simulink model "three_planar_robot"  (R2023a)
settings: Solver=VariableStepAuto  StartTime=0.0  StopTime=10.0  RelTol=1e-3
undefined symbols (not defined in the file or in its folder): DisplayRobot3
settings Model: Creator=LENOVO  LastModifiedBy=LENOVO

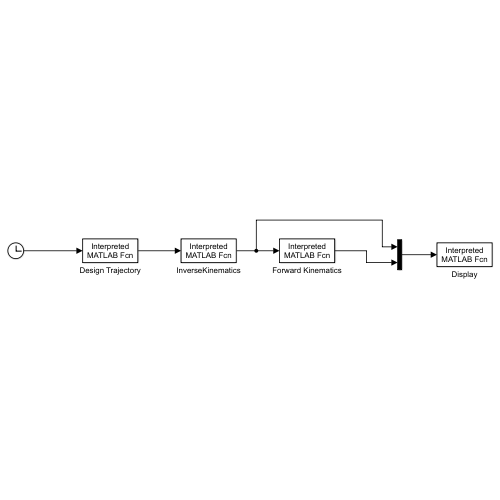
[thumbnail: Simulink's stored preview of the top-level diagram]
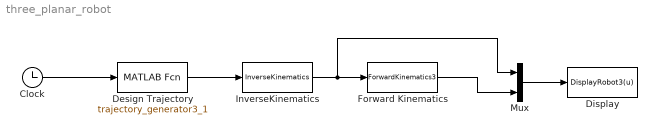
== system three_planar_robot ==
  Clock : Clock
  Design Trajectory : MATLABFcn  MATLABFcn=trajectory_generator3_1  OutputDimensions=2
  Display : MATLABFcn  MATLABFcn=DisplayRobot3(u)  OutputDimensions=0
  Forward Kinematics : MATLABFcn  MATLABFcn=ForwardKinematics3  OutputDimensions=2
  InverseKinematics : MATLABFcn  MATLABFcn=InverseKinematics  OutputDimensions=3
  Mux : Mux  Inputs=2
  wires:
  Design Trajectory/1 -> InverseKinematics/1
  Clock/1 -> Design Trajectory/1
  InverseKinematics/1 -> Mux/1, Forward Kinematics/1
  Forward Kinematics/1 -> Mux/2
  Mux/1 -> Display/1
